simulink model "X31dynamics_03_controller_GainS_MG_old"  (R2014b)
settings: Solver=ode45  StartTime=0.0  StopTime=30  FixedStep=0.01  RelTol=1e-3
InitFcn:
  | X31dynamics_03_controller_GainS_MG_init
values from neighbouring files (symbols this model uses):
  X31_controller = evalin('base','X31_controller')    [X31dynamics_03_controller_MG_iter_3_2_9_10.m]
undefined symbols (not defined in the file or in its folder): sigbuilder_block, X31_initC, X31_MnvrGen
libraries: simulink x9, QuaternionLib x5
settings Model: Creator=Ewing  LastModifiedBy=5909
settings SolverCC: AlgebraicLoopSolver=LineSearch
settings DataIOCC: SaveOutput=off  SaveTime=off
settings OptimizationCC: InlineParams=on  InlineInvariantSignals=on  EfficientFloat2IntCast=on
settings DebuggingCC: UnderspecifiedInitializationDetection=Classic  MergeDetectMultiDrivingBlocksExec=none  UniqueDataStoreMsg=error  StateNameClashWarn=warning
settings ModelReferenceCC: ModelReferencePassRootInputsByReference=off

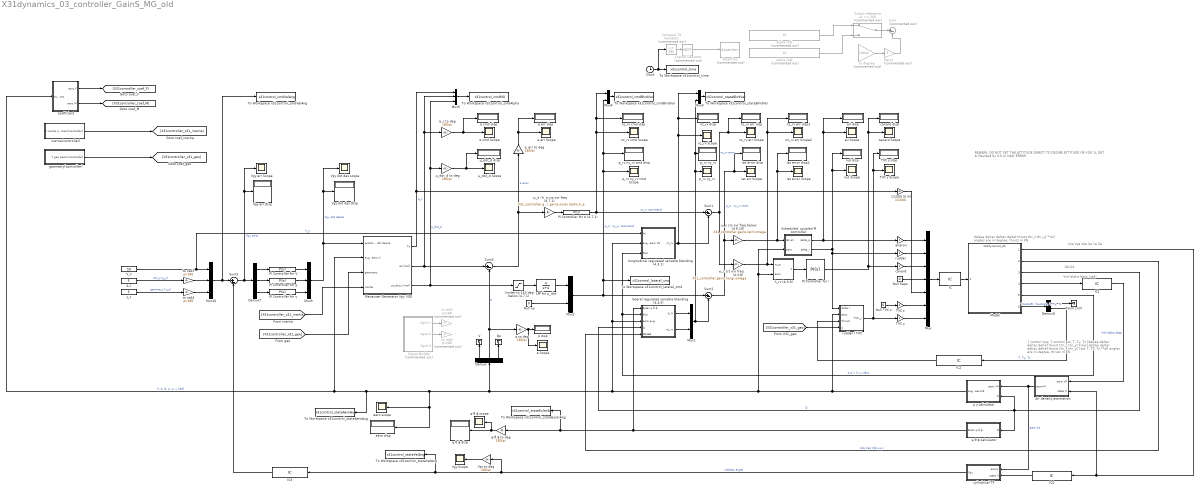
== system X31dynamics_03_controller_GainS_MG_old ==
  note: REMARK: DO NOT SET THE ATTITUDE DIRECT TO DESIRE ATTITUDE
      | OR YOU"LL GET A 'Devided by 0.0 or NaN' ERROR
  note: Q0-Q3
  note: Vxe Vye Vze
      | Xe   Ye   Ze
  note: deltaa deltar deltac deltaf thrust thr_z thr_y]
      | **all angles are in degree, thrust in KN
  note: Vinf alpha beta (rad)
  note: 7 contorl raw, 7 control act, T, Ty, Tz
      | [deltaa deltar deltac deltaf thrust thr_z thr_y] 7raw
      | [deltaa deltar deltac deltaf thrust thr_z thr_y] 7act
      | T, Ty, Tz
      | **all angles are in degree, thrust in KN
  1/1000 (K N) : Gain  Gain=1/1000
  Air density estimation : Subsystem
  Assertion : Assertion  Commented=on  AssertionFailFcn=|  StopWhenAssertionFail=off
      | set_param(bdroot,'SimulationCommand','pause'),
      | disp(sprintf('\nSimulation paused.'))
  Clock : Clock
  Compare To Constant : simulink/Logic and Bit Operations/Compare To Constant  Commented=on  relop=>=  const=180  OutDataTypeStr=boolean
  Demux : Demux  Outputs=[1 1 4]
  Demux7 : Demux  Outputs=3
  Demux9 : Demux  Outputs=[14 3]
  Gain1 : Gain  Commented=on  Gain=3
  IC : InitialCondition  Value=[ 0.0001 0.0001 00001 0 X31_initC.thrust 0 0.0001]
  IC1 : InitialCondition  Value=[50 0.01 0.01]
  IC2 : InitialCondition  Value=[X31_initC.thrust 0.00001 0]
  IC3 : InitialCondition  Value=[50 0 0]
  IC4 : InitialCondition  Value=[50 0 0 0.1 0.1 -0.1]
  LPF for μ_dot : TransferFcn  Numerator=[4]  Denominator=[1 4]
  Logical Operator : Logic  Commented=on  Operator=NOT  AllPortsSameDT=off  OutDataTypeStr=boolean
  Maneuver Generator Vχγ  NDI : Subsystem
  Model : ModelReference  ModelNameDialog=X31dynamics_03.slx  SimulationMode=Normal  ModelReferenceVersion=1.302  CopyOfModelName=X31dynamics_03.slx  DefaultDataLogging=on
  Mux : Mux  Inputs=7
  Mux{1..4} (4 alike) : Mux  Inputs=2
  Mux10 : Mux  Inputs=3
  Mux5 : Mux  Inputs=3
  Mux9 : Mux  Inputs=3
  Null TVC z : Constant  Value=0
  Null flaps : Constant  Value=0
  Null ny : Constant  Value=0
  PI Controller for V : simulink/Continuous/PID Controller  Controller=PI  TimeDomain=Continuous-time  SampleTime=-1  IntegratorMethod=Forward Euler  FilterMethod=Forward Euler  Form=Parallel  P=X31_MnvrGen.gains.vel.P_gain  I=X31_MnvrGen.gains.vel.I_gain  D=0  N=100  InitialConditionSource=internal  InitialConditionForIntegrator=0  InitialConditionForFilter=0  ExternalReset=none  LimitOutput=off  UpperSaturationLimit=inf  LowerSaturationLimit=-inf  LinearizeAsGain=on  AntiWindupMode=none  Kb=1  TrackingMode=off  Kt=1  PParamMin=[]  PParamMax=[]  IParamMin=[]  IParamMax=[]  DParamMin=[]  DParamMax=[]  NParamMin=[]  NParamMax=[]  KbParamMin=[]  KbParamMax=[]  KtParamMin=[]  KtParamMax=[]  POutMin=[]  POutMax=[]  IOutMin=[]  IOutMax=[]  DOutMin=[]  DOutMax=[]  NOutMin=[]  NOutMax=[]  KbOutMin=[]  KbOutMax=[]  KtOutMin=[]  KtOutMax=[]  IntegratorOutMin=[]  IntegratorOutMax=[]  FilterOutMin=[]  FilterOutMax=[]  SumOutMin=[]  SumOutMax=[]  SumI1OutMin=[]  SumI1OutMax=[]  SumI2OutMin=[]  SumI2OutMax=[]  SumI3OutMin=[]  SumI3OutMax=[]  SumDOutMin=[]  SumDOutMax=[]  SaturationOutMin=[]  SaturationOutMax=[]  IntegratorContinuousStateAttributes=''  IntegratorStateMustResolveToSignalObject=off  IntegratorRTWStateStorageClass=Auto  FilterContinuousStateAttributes=''  FilterStateMustResolveToSignalObject=off  FilterRTWStateStorageClass=Auto  DifferentiatorICPrevScaledInput=0  DifferentiatorOutMin=[]  DifferentiatorOutMax=[]  UseFilter=on
  PI Controller for r : simulink/Continuous/PID Controller  Controller=PI  TimeDomain=Continuous-time  SampleTime=-1  IntegratorMethod=Forward Euler  FilterMethod=Forward Euler  Form=Parallel  P=X31_controller.gains.longi.P_gain  I=X31_controller.gains.longi.I_gain  D=0  N=100  InitialConditionSource=internal  InitialConditionForIntegrator=0  InitialConditionForFilter=0  ExternalReset=none  LimitOutput=off  UpperSaturationLimit=inf  LowerSaturationLimit=-inf  LinearizeAsGain=on  AntiWindupMode=none  Kb=1  TrackingMode=off  Kt=1  PParamMin=[]  PParamMax=[]  IParamMin=[]  IParamMax=[]  DParamMin=[]  DParamMax=[]  NParamMin=[]  NParamMax=[]  KbParamMin=[]  KbParamMax=[]  KtParamMin=[]  KtParamMax=[]  POutMin=[]  POutMax=[]  IOutMin=[]  IOutMax=[]  DOutMin=[]  DOutMax=[]  NOutMin=[]  NOutMax=[]  KbOutMin=[]  KbOutMax=[]  KtOutMin=[]  KtOutMax=[]  IntegratorOutMin=[]  IntegratorOutMax=[]  FilterOutMin=[]  FilterOutMax=[]  SumOutMin=[]  SumOutMax=[]  SumI1OutMin=[]  SumI1OutMax=[]  SumI2OutMin=[]  SumI2OutMax=[]  SumI3OutMin=[]  SumI3OutMax=[]  SumDOutMin=[]  SumDOutMax=[]  SaturationOutMin=[]  SaturationOutMax=[]  IntegratorContinuousStateAttributes=''  IntegratorStateMustResolveToSignalObject=off  IntegratorRTWStateStorageClass=Auto  FilterContinuousStateAttributes=''  FilterStateMustResolveToSignalObject=off  FilterRTWStateStorageClass=Auto  DifferentiatorICPrevScaledInput=0  DifferentiatorOutMin=[]  DifferentiatorOutMax=[]  UseFilter=on
  PI Controller for α (4.7.1) : simulink/Continuous/PID Controller  Controller=PI  TimeDomain=Continuous-time  SampleTime=-1  IntegratorMethod=Forward Euler  FilterMethod=Forward Euler  Form=Parallel  P=X31_controller.gains.outer.alpha.P_gain  I=X31_controller.gains.outer.alpha.I_gain  D=0  N=100  InitialConditionSource=internal  InitialConditionForIntegrator=0  InitialConditionForFilter=0  ExternalReset=none  LimitOutput=off  UpperSaturationLimit=inf  LowerSaturationLimit=-inf  LinearizeAsGain=on  AntiWindupMode=none  Kb=1  TrackingMode=off  Kt=1  PParamMin=[]  PParamMax=[]  IParamMin=[]  IParamMax=[]  DParamMin=[]  DParamMax=[]  NParamMin=[]  NParamMax=[]  KbParamMin=[]  KbParamMax=[]  KtParamMin=[]  KtParamMax=[]  POutMin=[]  POutMax=[]  IOutMin=[]  IOutMax=[]  DOutMin=[]  DOutMax=[]  NOutMin=[]  NOutMax=[]  KbOutMin=[]  KbOutMax=[]  KtOutMin=[]  KtOutMax=[]  IntegratorOutMin=[]  IntegratorOutMax=[]  FilterOutMin=[]  FilterOutMax=[]  SumOutMin=[]  SumOutMax=[]  SumI1OutMin=[]  SumI1OutMax=[]  SumI2OutMin=[]  SumI2OutMax=[]  SumI3OutMin=[]  SumI3OutMax=[]  SumDOutMin=[]  SumDOutMax=[]  SaturationOutMin=[]  SaturationOutMax=[]  IntegratorContinuousStateAttributes=''  IntegratorStateMustResolveToSignalObject=off  IntegratorRTWStateStorageClass=Auto  FilterContinuousStateAttributes=''  FilterStateMustResolveToSignalObject=off  FilterRTWStateStorageClass=Auto  DifferentiatorICPrevScaledInput=0  DifferentiatorOutMin=[]  DifferentiatorOutMax=[]  UseFilter=on
  PI Controller for γ : simulink/Continuous/PID Controller  Controller=PI  TimeDomain=Continuous-time  SampleTime=-1  IntegratorMethod=Forward Euler  FilterMethod=Forward Euler  Form=Parallel  P=X31_MnvrGen.gains.gamma.P_gain  I=X31_MnvrGen.gains.gamma.P_gain  D=0  N=100  InitialConditionSource=internal  InitialConditionForIntegrator=0  InitialConditionForFilter=0  ExternalReset=none  LimitOutput=off  UpperSaturationLimit=inf  LowerSaturationLimit=-inf  LinearizeAsGain=on  AntiWindupMode=none  Kb=1  TrackingMode=off  Kt=1  PParamMin=[]  PParamMax=[]  IParamMin=[]  IParamMax=[]  DParamMin=[]  DParamMax=[]  NParamMin=[]  NParamMax=[]  KbParamMin=[]  KbParamMax=[]  KtParamMin=[]  KtParamMax=[]  POutMin=[]  POutMax=[]  IOutMin=[]  IOutMax=[]  DOutMin=[]  DOutMax=[]  NOutMin=[]  NOutMax=[]  KbOutMin=[]  KbOutMax=[]  KtOutMin=[]  KtOutMax=[]  IntegratorOutMin=[]  IntegratorOutMax=[]  FilterOutMin=[]  FilterOutMax=[]  SumOutMin=[]  SumOutMax=[]  SumI1OutMin=[]  SumI1OutMax=[]  SumI2OutMin=[]  SumI2OutMax=[]  SumI3OutMin=[]  SumI3OutMax=[]  SumDOutMin=[]  SumDOutMax=[]  SaturationOutMin=[]  SaturationOutMax=[]  IntegratorContinuousStateAttributes=''  IntegratorStateMustResolveToSignalObject=off  IntegratorRTWStateStorageClass=Auto  FilterContinuousStateAttributes=''  FilterStateMustResolveToSignalObject=off  FilterRTWStateStorageClass=Auto  DifferentiatorICPrevScaledInput=0  DifferentiatorOutMin=[]  DifferentiatorOutMax=[]  UseFilter=on
  PI Controller for χ : simulink/Continuous/PID Controller  Controller=PI  TimeDomain=Continuous-time  SampleTime=-1  IntegratorMethod=Forward Euler  FilterMethod=Forward Euler  Form=Parallel  P=X31_MnvrGen.gains.chi.P_gain  I=X31_MnvrGen.gains.chi.I_gain  D=0  N=100  InitialConditionSource=internal  InitialConditionForIntegrator=0  InitialConditionForFilter=0  ExternalReset=none  LimitOutput=off  UpperSaturationLimit=inf  LowerSaturationLimit=-inf  LinearizeAsGain=on  AntiWindupMode=none  Kb=1  TrackingMode=off  Kt=1  PParamMin=[]  PParamMax=[]  IParamMin=[]  IParamMax=[]  DParamMin=[]  DParamMax=[]  NParamMin=[]  NParamMax=[]  KbParamMin=[]  KbParamMax=[]  KtParamMin=[]  KtParamMax=[]  POutMin=[]  POutMax=[]  IOutMin=[]  IOutMax=[]  DOutMin=[]  DOutMax=[]  NOutMin=[]  NOutMax=[]  KbOutMin=[]  KbOutMax=[]  KtOutMin=[]  KtOutMax=[]  IntegratorOutMin=[]  IntegratorOutMax=[]  FilterOutMin=[]  FilterOutMax=[]  SumOutMin=[]  SumOutMax=[]  SumI1OutMin=[]  SumI1OutMax=[]  SumI2OutMin=[]  SumI2OutMax=[]  SumI3OutMin=[]  SumI3OutMax=[]  SumDOutMin=[]  SumDOutMax=[]  SaturationOutMin=[]  SaturationOutMax=[]  IntegratorContinuousStateAttributes=''  IntegratorStateMustResolveToSignalObject=off  IntegratorRTWStateStorageClass=Auto  FilterContinuousStateAttributes=''  FilterStateMustResolveToSignalObject=off  FilterRTWStateStorageClass=Auto  DifferentiatorICPrevScaledInput=0  DifferentiatorOutMin=[]  DifferentiatorOutMax=[]  UseFilter=on
  "Scheduled, coupled PI controller" : Subsystem
  Signal Builder : Subsystem  Tag=STV Subsys  Commented=on  LoadFcn=sigbuilder_block('load');  StartFcn=sigbuilder_block('start');  StopFcn=sigbuilder_block('stop');  ClipboardFcn=sigbuilder_block('clipboard');  mask(Sigbuilder block){}
      mask help: Simulink:masks:SigbuilderBlock_MD
      mask init:
      | if ~strcmp(get_param(bdroot(gcbh),'SimulationStatus'),'stopped') tuvar = sigbuilder_block('maskInit'); end
      settings: CopyFcn=sigbuilder_block('copy');  DeleteFcn=sigbuilder_block('delete');  ModelCloseFcn=sigbuilder_block('modelClose');  PreSaveFcn=sigbuilder_block('preSave');  PauseFcn=sigbuilder_block('pause');  ContinueFcn=sigbuilder_block('continue');  NameChangeFcn=sigbuilder_block('namechange');  OpenFcn=sigbuilder_block('open',[437.6 199.2 550.4 400 ]);  CloseFcn=sigbuilder_block('close');
      mask Display: plot(0, 0, 100, 100,[2, 2, 32, 32, 2], [68, 8, 8, 68, 68],[32, 2], [38, 38], [32, 19, 2],[53, 60, 44], [32, 17, 17, 2],[16, 16, 31, 31]);txt = getActiveGroup(gcbh);text(2, 100, txt,'verticalAlignment', 'top');
  Sum : Sum  Commented=on  Inputs=|+-
  Sum{1..3,5} (4 alike) : Sum  Inputs=|+-
  Switch reference : Switch  Commented=on  Threshold=200
  TVC y : Gain
  TVC y Scope : Scope
      settings: SaveName=ScopeData13
  TVC y disp : Display
  TVC z : Gain
  Term cntrl : Terminator
  To Workspace x31control_cmdAlpha : ToWorkspace  VariableName=x31control_cmdMG  SaveFormat=Timeseries  SampleTime=-1
  To Workspace x31control_cmdBlndVar : ToWorkspace  VariableName=x31control_cmdBlndVar  SaveFormat=Timeseries  SampleTime=-1
  To Workspace x31control_cmdVelAng : ToWorkspace  VariableName=x31control_cmdVelAng  SaveFormat=Timeseries  SampleTime=-1
  To Workspace x31control_lateral_cmd : ToWorkspace  VariableName=x31control_lateral_cmd  SaveFormat=Timeseries  SampleTime=-1
  To Workspace x31control_stateAeroAug : ToWorkspace  VariableName=x31control_stateAeroAug  SaveFormat=Timeseries  SampleTime=-1
  To Workspace x31control_stateBlndVar : ToWorkspace  VariableName=x31control_stateBlndVar  SaveFormat=Timeseries  SampleTime=-1
  To Workspace x31control_stateEulerAng : ToWorkspace  VariableName=x31control_stateEulerAng  SaveFormat=Timeseries  SampleTime=-1
  To Workspace x31control_stateVelAng : ToWorkspace  VariableName=x31control_stateVelAng  SaveFormat=Timeseries  SampleTime=-1
  To Workspace x31control_time : ToWorkspace  VariableName=x31control_time  SaveFormat=Timeseries  SampleTime=-1
  V : Terminator
  V_c : Constant  Value=50
  Vχγ Scope : Scope
      settings: ShowLegends=on  TimeRange=30  YMin=-1000  YMax=6000  SaveName=ScopeData18
  Vχγ dot des Disp : Display
  Vχγ dot des scope : Scope
      settings: TickLabels=on  ShowLegends=on  SaveName=ScopeData15
  Vχγ err Disp : Display
  Vχγ err Scope : Scope
      settings: TimeRange=3.005065038857998  YMin=2.02995391705069  YMax=6.02995391705069  SaveName=ScopeData14
  Vχγ to deg : Gain  Gain=180/pi
  aero disp : Display
  aero scope : Scope
      settings: ShowLegends=on  YMin=-1000  YMax=6000  SaveName=ScopeData8
  ail Scope : Scope
      settings: SaveName=ScopeData11
  ail disp : Display
  aileron : Gain
  alpha ref1 : Constant  Commented=on  Value=10
  alpha ref2 : Constant  Commented=on  Value=10
  canard : Gain
  canard Scope : Scope
      settings: SaveName=ScopeData12
  canard disp : Display
  coefficient : Subsystem
  cylindrical TF : Subsystem
  geometry(controller) : Subsystem
  h_rv (4.3.9) : Subsystem
  inertia(controller) : Subsystem
  lat err Scope : Scope
      settings: SaveName=ScopeData5
  lat error Scope : Scope
      settings: SaveName=ScopeData9
  lat error disp : Display
  lat error disp2 : Display
  lateral regulated variable blending (4.4.5) : Subsystem
  limiter to 143 deg below (4.7.1) : Saturate  UpperLimit=143 * pi / 180  LowerLimit=-143 * pi / 180
  longitudinal regulated variable blending (4.3.1) : Subsystem
  nz_rv Scope : Scope
      settings: SaveName=ScopeData16
  nz_rv cmd Scope : Scope
      settings: SaveName=ScopeData2
  nz_rv cmd disp : Display
  nz_rv disp : Display
  nz_rv err Scope : Scope
      settings: SaveName=ScopeData7
  nz_rv err Scope2 : Scope
      settings: SaveName=ScopeData10
  nz_rv err disp : Display
  nz_rv err disp2 : Display
  p_rv ny_rv : Display
  "p_rv ny_rv " : Scope
      settings: SaveName=ScopeData6
  p_rv ny_rv cmd Scope : Scope
      settings: SaveName=ScopeData4
  p_rv ny_rv cmd disp : Display
  rud Scope : Scope
      settings: SaveName=ScopeData17
  rud disp : Display
  rudder : Gain
  rudder / TVC : Subsystem
  to degree : Gain  Commented=on  Gain=180/pi
  to rad1 : Gain  Commented=on  Gain=pi/180
  to rad2 : Gain  Commented=on  Gain=pi/180
  to rad3 : Gain  Gain=pi/180
  to rad4 : Gain  Gain=pi/180
  α Scope : Scope
      settings: SaveName=ScopeData20
  α cmd Scope : Scope
  α cmd disp : Display
  α disp : Display
  α err Scope : Scope
  α err disp : Display
  α to deg : Gain  Gain=180/pi
  α_c to deg : Gain  Gain=180/pi
  α_err to deg : Gain  Gain=180/pi
  βρ : Terminator
  γ_c : Constant  Value=5
  μ γ calculator : Subsystem
  μ_dot_d Scope : Scope
      settings: SaveName=ScopeData3
  μ_dot_d disp : Display
  μ_dot_d to deg : Gain  Gain=180/pi
  χ_c : Constant  Value=5
  ψ θ ϕ calculator : Subsystem
  ψ θ ϕ disp : Display
  ψ θ ϕ scope : Scope
      settings: ShowLegends=on  TimeRange=30  YMin=-20  YMax=160  SaveName=ScopeData19
  ψ θ ϕ to deg : Gain  Gain=180/pi
  ω_a / h_a crs ovr freq (4.7.1) : Gain  Gain=X31_controller.gains.outer.alpha.omega / X31_controller.gains.outer.alpha.h_a
  ω_c crs ovr freq (4.3.8) : Gain  Gain=X31_controller.gains.longi.omega
  ω_c crs ovr freq below (4.6.10) : Gain  Gain=X31_controller.gains.latrl.omega
  wires:
  Null flaps/1 -> Mux/4
  rudder/1 -> Mux/2
  canard/1 -> Mux/3
  Mux/1 -> IC/1
  IC/1 -> Model/1
  alpha ref1/1 -> Switch reference/1
  alpha ref2/1 -> Switch reference/3
  Clock/1 -> Compare To Constant/1, To Workspace x31control_time/1
  aileron/1 -> Mux/1
  Model/4 -> IC1/1
  Switch reference/1 -> Sum/1
  to degree/1 -> Gain1/1
  Maneuver Generator Vχγ  NDI/1(Tc) -> Mux5/1, 1/1000 (K N)/1
  Gain1/1 -> Sum/2
  TVC z/1 -> Mux/6
  TVC y/1 -> Mux/7
  [X31controller_x31_geo] -> rudder / TVC/4(geometry)
  Null TVC z/1 -> TVC z/1
  rudder / TVC/1(TVC_y) -> TVC y/1, TVC y Scope/1, TVC y disp/1
  Sum1/1 -> ω_c crs ovr freq (4.3.8)/1, nz_rv err disp/1, nz_rv err Scope/1  "nz_rv error"
  Model/2 -> lateral regulated variable blending (4.4.5)/5(stateB)  "Vxb Vyb Vzb p q r"
  coefficient/1(aero F) -> [X31controller_coef_F]
  coefficient/2(aero M) -> [X31controller_coef_M]
  Maneuver Generator Vχγ  NDI/2(αc (rad)) -> α_c to deg/1, Mux5/2, Sum3/1  "α_c"
  μ γ calculator/1(aug. aeroV6) -> To Workspace x31control_stateAeroAug/1, coefficient/1(aug. aero), Maneuver Generator Vχγ  NDI/2(aug. aero V), aero scope/1, aero disp/1, Demux/1, longitudinal regulated variable blending (4.3.1)/2(aug. aero V6), lateral regulated variable blending (4.4.5)/3(aero aug.), "Scheduled, coupled PI controller"/2(aero), h_rv (4.3.9)/2(aero), rudder / TVC/2(aero)  "V, α, β, ρ, μ, γ (rad)"
  Sum3/1 -> α_err to deg/1, ω_a / h_a crs ovr freq (4.7.1)/1  "α error"
  Maneuver Generator Vχγ  NDI/3(μc_dot_c (rad)) -> μ_dot_d to deg/1, Mux5/3, limiter to 143 deg below (4.7.1)/1  "μ_dot_d"
  Model/3 -> ψ θ ϕ calculator/1(Q), lateral regulated variable blending (4.4.5)/4(Q), μ γ calculator/2(Q)  "Q"
  Demux9/2 -> IC2/1  "T, Ty, Tz"
  Demux/1 -> V/1
  Demux/3 -> βρ/1
  IC1/1 -> Air density estimation/1(aero V3)  "Vinf alpha beta"
  Demux9/1 -> Term cntrl/1
  Model/6 -> Demux9/1  "7controR, 7controlA, T, Ty, Tz"
  Model/5 -> longitudinal regulated variable blending (4.3.1)/3(IMU), lateral regulated variable blending (4.4.5)/2(IMU)  "p q r, (x y z)acc"
  longitudinal regulated variable blending (4.3.1)/1(nz_rv) -> Sum1/2, nz_rv Scope/1, Mux3/1, nz_rv disp/1
  ω_c crs ovr freq (4.3.8)/1 -> h_rv (4.3.9)/1(nz_e), nz_rv err Scope2/1, nz_rv err disp2/1
  PI Controller for α (4.7.1)/1 -> Sum1/1, nz_rv cmd Scope/1, Mux4/1, nz_rv cmd disp/1  "nz_rv command"
  h_rv (4.3.9)/1(1 /h_rv) -> PI Controller for r/1
  ψ θ ϕ calculator/1(Eular ψ θ ϕ) -> To Workspace x31control_stateEulerAng/1, ψ θ ϕ to deg/1, lateral regulated variable blending (4.4.5)/1(Eular ψ θ ϕ)
  "Scheduled, coupled PI controller"/2(delta_r) -> rudder/1, rudder / TVC/1(delta r), rud disp/1, rud Scope/1
  lateral regulated variable blending (4.4.5)/1(p_rv) -> Mux1/1
  lateral regulated variable blending (4.4.5)/2(ny_rv) -> Mux1/2
  Mux2/1 -> Sum2/1, Mux4/2, p_rv ny_rv cmd disp/1, p_rv ny_rv cmd Scope/1, To Workspace x31control_lateral_cmd/1  "p_rv  ny_rv command"
  Mux1/1 -> Sum2/2, Mux3/2, p_rv ny_rv/1, "p_rv ny_rv "/1
  Sum2/1 -> lat error disp/1, lat err Scope/1, ω_c crs ovr freq below (4.6.10)/1  "p_rv  ny_rv error"
  ω_c crs ovr freq below (4.6.10)/1 -> "Scheduled, coupled PI controller"/1(lat err), lat error disp2/1, lat error Scope/1
  "Scheduled, coupled PI controller"/1(delta_a) -> ail disp/1, ail Scope/1, aileron/1
  Null ny/1 -> Mux2/2
  limiter to 143 deg below (4.7.1)/1 -> LPF for μ_dot/1
  ω_a / h_a crs ovr freq (4.7.1)/1 -> PI Controller for α (4.7.1)/1
  LPF for μ_dot/1 -> Mux2/1
  IC2/1 -> rudder / TVC/3(Thrust)
  geometry(controller)/1(7 geo param(controller)) -> [X31controller_x31_geo]
  inertia(controller)/1(7 inertia param(controller)) -> [X31controller_x31_inertia]
  Mux10/1 -> To Workspace x31control_cmdVelAng/1, Sum5/1
  Sum5/1 -> Demux7/1, Vχγ err Disp/1, Vχγ err Scope/1  "Vχγ error"
  Demux7/3 -> PI Controller for γ/1
  Demux7/2 -> PI Controller for χ/1
  Demux7/1 -> PI Controller for V/1
  PI Controller for γ/1 -> Mux9/3
  PI Controller for χ/1 -> Mux9/2
  PI Controller for V/1 -> Mux9/1
  Mux9/1 -> Maneuver Generator Vχγ  NDI/1(positionVχγ dot desire), Vχγ dot des scope/1, Vχγ dot des Disp/1  "Vχγ dot desire"
  V_c/1 -> longitudinal regulated variable blending (4.3.1)/1(Vc), Mux10/1  "V_c"
  χ_c/1 -> to rad3/1  "Chi_c (χ_c)"
  γ_c/1 -> to rad4/1  "gamma_c (γ_c)"
  to rad3/1 -> Mux10/2
  to rad4/1 -> Mux10/3
  Air density estimation/1(aeroV4) -> cylindrical TF/1(aeroV), μ γ calculator/1(aero V4)  "aero V4"
  cylindrical TF/1(Vχγ) -> To Workspace x31control_stateVelAng/1, IC3/1, Vχγ to deg/1  "velocity angle"
  Model/1 -> Air density estimation/2(state X), IC4/1
  Demux/2 -> Sum3/2, α to deg/1  "α"
  IC3/1 -> Sum5/2
  IC4/1 -> cylindrical TF/2(state X)
  PI Controller for r/1 -> canard Scope/1, canard disp/1, canard/1
  1/1000 (K N)/1 -> Mux/5
  Compare To Constant/1 -> Logical Operator/1
  Logical Operator/1 -> Assertion/1
  ψ θ ϕ to deg/1 -> ψ θ ϕ disp/1, ψ θ ϕ scope/1
  Vχγ to deg/1 -> Vχγ Scope/1
  [X31controller_x31_geo] -> Maneuver Generator Vχγ  NDI/3(geometry)
  [X31controller_x31_inertia] -> Maneuver Generator Vχγ  NDI/4(inertia)
  α to deg/1 -> α Scope/1, α disp/1
  Signal Builder/1(Signal 1) -> to rad1/1
  Signal Builder/2(Signal 2) -> to rad2/1
  α_c to deg/1 -> α cmd Scope/1, α cmd disp/1
  μ_dot_d to deg/1 -> μ_dot_d Scope/1, μ_dot_d disp/1
  Mux3/1 -> To Workspace x31control_stateBlndVar/1
  Mux4/1 -> To Workspace x31control_cmdBlndVar/1
  α_err to deg/1 -> α err disp/1, α err Scope/1
  Mux5/1 -> To Workspace x31control_cmdAlpha/1

== system X31dynamics_03_controller_GainS_MG_old/Air density estimation ==
  aero V3 : Inport
  state X : Inport  Port=2
  Mux : Mux  Inputs=2
  Terminator : Terminator
  air_density : Constant  Value=1.23
  aeroV4 : Outport
  wires:
  aero V3/1 -> Mux/1
  Mux/1 -> aeroV4/1
  air_density/1 -> Mux/2
  state X/1 -> Terminator/1

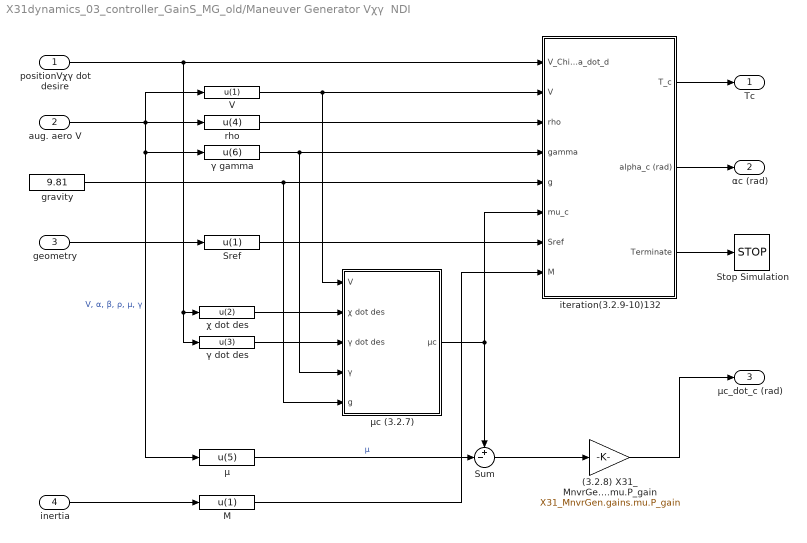
== system X31dynamics_03_controller_GainS_MG_old/Maneuver Generator Vχγ  NDI ==
  positionVχγ dot desire : Inport
  aug. aero V : Inport  Port=2
  geometry : Inport  Port=3
  inertia : Inport  Port=4
  (3.2.8) X31_MnvrGen.gains.mu.P_gain : Gain  Gain=X31_MnvrGen.gains.mu.P_gain
  M : Fcn  Expr=u(1)
  Sref : Fcn  Expr=u(1)
  Stop Simulation : Stop
  Sum : Sum  Inputs=+-|
  V : Fcn  Expr=u(1)
  gravity : Constant  Value=9.81
  iteration(3.2.9-10)132 : Subsystem
  rho : Fcn  Expr=u(4)
  γ dot des : Fcn  Expr=u(3)
  γ gamma : Fcn  Expr=u(6)
  μ : Fcn  Expr=u(5)
  μc (3.2.7) : Subsystem
  χ dot des : Fcn  Expr=u(2)
  Tc : Outport
  αc (rad) : Outport  Port=2
  μc_dot_c (rad) : Outport  Port=3
  wires:
  positionVχγ dot desire/1 -> γ dot des/1, χ dot des/1, iteration(3.2.9-10)132/1(V_Chi_Gamma_dot_d)
  aug. aero V/1 -> μ/1, γ gamma/1, V/1, rho/1  "V, α, β, ρ, μ, γ"
  μc (3.2.7)/1(μc) -> iteration(3.2.9-10)132/6(mu_c), Sum/1
  μ/1 -> Sum/2  "μ"
  Sum/1 -> (3.2.8) X31_MnvrGen.gains.mu.P_gain/1
  (3.2.8) X31_MnvrGen.gains.mu.P_gain/1 -> μc_dot_c (rad)/1
  iteration(3.2.9-10)132/2(alpha_c (rad)) -> αc (rad)/1
  iteration(3.2.9-10)132/1(T_c) -> Tc/1
  geometry/1 -> Sref/1
  inertia/1 -> M/1
  V/1 -> μc (3.2.7)/1(V), iteration(3.2.9-10)132/2(V)
  γ dot des/1 -> μc (3.2.7)/3(γ dot des)
  χ dot des/1 -> μc (3.2.7)/2(χ dot des)
  gravity/1 -> μc (3.2.7)/5(g), iteration(3.2.9-10)132/5(g)
  γ gamma/1 -> μc (3.2.7)/4(γ), iteration(3.2.9-10)132/4(gamma)
  rho/1 -> iteration(3.2.9-10)132/3(rho)
  iteration(3.2.9-10)132/3(Terminate) -> Stop Simulation/1
  Sref/1 -> iteration(3.2.9-10)132/7(Sref)
  M/1 -> iteration(3.2.9-10)132/8(M)

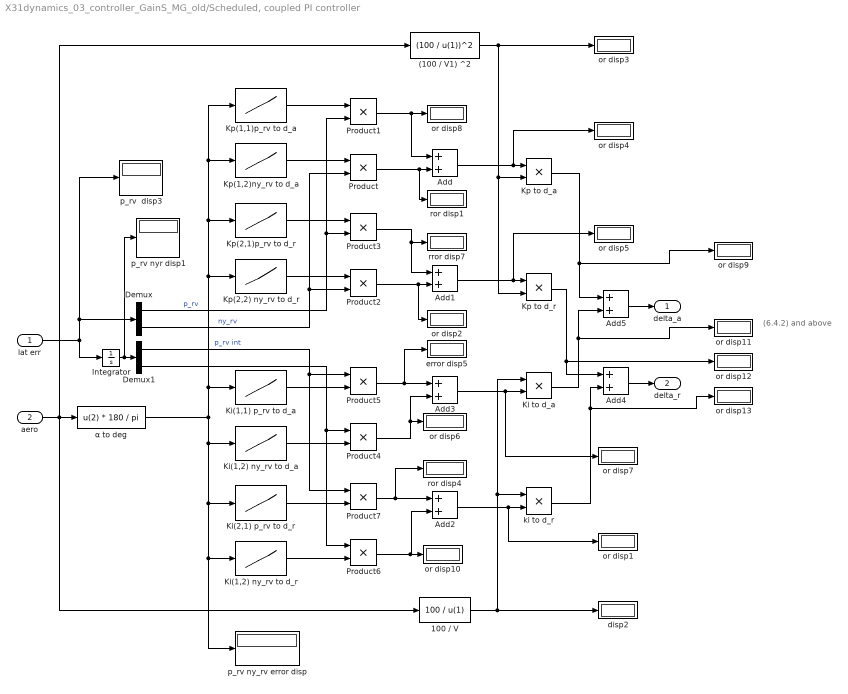
== system X31dynamics_03_controller_GainS_MG_old/Scheduled, coupled PI controller ==
  note: (6.4.2) and above
  lat err : Inport
  aero : Inport  Port=2
  " error disp5" : Display
  (100 / V1) ^2 : Fcn  Expr=(100 / u(1))^2
  100 / V : Fcn  Expr=100 / u(1)
  Add{,1..5} (6 alike) : Sum
  Demux : Demux  Outputs=2
  Demux1 : Demux  Outputs=2
  Integrator : Integrator
  Ki to d_a : Product
  Ki(1,1) p_rv to d_a : Lookup_n-D  NumberOfTableDimensions=1  BreakpointsForDimension1=X31_controller.gains.latrl.I_gain.mat1_1.alpha  Table=X31_controller.gains.latrl.I_gain.mat1_1.gain  ExtrapMethod=Clip  UseLastTableValue=on  InternalRulePriority=Speed  RndMeth=Simplest  InputSameDT=on
  Ki(1,2) ny_rv to d_a : Lookup_n-D  NumberOfTableDimensions=1  BreakpointsForDimension1=X31_controller.gains.latrl.I_gain.mat1_2.alpha  Table=X31_controller.gains.latrl.I_gain.mat1_2.gain  ExtrapMethod=Clip  UseLastTableValue=on  InternalRulePriority=Speed  RndMeth=Simplest  InputSameDT=on
  Ki(1,2) ny_rv to d_r : Lookup_n-D  NumberOfTableDimensions=1  BreakpointsForDimension1=X31_controller.gains.latrl.I_gain.mat2_2.alpha  Table=X31_controller.gains.latrl.I_gain.mat2_2.gain  ExtrapMethod=Clip  UseLastTableValue=on  InternalRulePriority=Speed  RndMeth=Simplest  InputSameDT=on
  Ki(2,1) p_rv to d_r : Lookup_n-D  NumberOfTableDimensions=1  BreakpointsForDimension1=X31_controller.gains.latrl.I_gain.mat2_1.alpha  Table=X31_controller.gains.latrl.I_gain.mat2_1.gain  ExtrapMethod=Clip  UseLastTableValue=on  InternalRulePriority=Speed  RndMeth=Simplest  InputSameDT=on
  Kp to d_a : Product
  Kp to d_r : Product
  Kp(1,1)p_rv to d_a : Lookup_n-D  NumberOfTableDimensions=1  BreakpointsForDimension1=X31_controller.gains.latrl.P_gain.mat1_1.alpha  Table=X31_controller.gains.latrl.P_gain.mat1_1.gain  ExtrapMethod=Clip  UseLastTableValue=on  InternalRulePriority=Speed  RndMeth=Simplest  InputSameDT=on
  Kp(1,2)ny_rv to d_a : Lookup_n-D  NumberOfTableDimensions=1  BreakpointsForDimension1=X31_controller.gains.latrl.P_gain.mat1_2.alpha  Table=X31_controller.gains.latrl.P_gain.mat1_2.gain  ExtrapMethod=Clip  UseLastTableValue=on  InternalRulePriority=Speed  RndMeth=Simplest  InputSameDT=on
  Kp(2,1)p_rv to d_r : Lookup_n-D  NumberOfTableDimensions=1  BreakpointsForDimension1=X31_controller.gains.latrl.P_gain.mat2_1.alpha  Table=X31_controller.gains.latrl.P_gain.mat2_1.gain  ExtrapMethod=Clip  UseLastTableValue=on  InternalRulePriority=Speed  RndMeth=Simplest  InputSameDT=on
  Kp(2,2) ny_rv to d_r : Lookup_n-D  NumberOfTableDimensions=1  BreakpointsForDimension1=X31_controller.gains.latrl.P_gain.mat2_2.alpha  Table=X31_controller.gains.latrl.P_gain.mat2_2.gain  ExtrapMethod=Clip  UseLastTableValue=on  InternalRulePriority=Speed  RndMeth=Simplest  InputSameDT=on
  Product{,1..7} (8 alike) : Product
  disp2 : Display
  ki to d_r : Product
  or disp{1..13} (13 alike) : Display
  p_rv  disp3 : Display
  p_rv ny_rv error disp : Display
  p_rv nyr disp1 : Display
  ror disp1 : Display
  ror disp4 : Display
  rror disp7 : Display
  α to deg : Fcn  Expr=u(2) * 180 / pi
  delta_a : Outport
  delta_r : Outport  Port=2
  wires:
  lat err/1 -> p_rv  disp3/1, Demux/1, Integrator/1
  Demux/2 -> Product/2, Product2/2  "ny_rv"
  Integrator/1 -> p_rv nyr disp1/1, Demux1/1
  Demux1/1 -> Product7/1, Product5/1  "p_rv int"
  Demux1/2 -> Product6/1, Product4/1
  aero/1 -> 100 / V/1, (100 / V1) ^2/1, α to deg/1
  Demux/1 -> Product1/2, Product3/2  "p_rv"
  Kp(1,2)ny_rv to d_a/1 -> Product/1
  Kp(1,1)p_rv to d_a/1 -> Product1/1
  Kp(2,1)p_rv to d_r/1 -> Product3/1
  Kp(2,2) ny_rv to d_r/1 -> Product2/1
  Ki(1,2) ny_rv to d_r/1 -> Product6/2
  Ki(2,1) p_rv to d_r/1 -> Product7/2
  Ki(1,1) p_rv to d_a/1 -> Product5/2
  α to deg/1 -> p_rv ny_rv error disp/1, Ki(1,2) ny_rv to d_r/1, Ki(2,1) p_rv to d_r/1, Ki(1,2) ny_rv to d_a/1, Kp(2,1)p_rv to d_r/1, Kp(1,1)p_rv to d_a/1, Kp(1,2)ny_rv to d_a/1, Kp(2,2) ny_rv to d_r/1, Ki(1,1) p_rv to d_a/1
  Product1/1 -> or disp8/1, Add/1
  Product/1 -> ror disp1/1, Add/2
  Product3/1 -> Add1/1, rror disp7/1
  Product2/1 -> or disp2/1, Add1/2
  Product5/1 -> Add3/1, " error disp5"/1
  Product7/1 -> Add2/1, ror disp4/1
  Product6/1 -> Add2/2, or disp10/1
  100 / V/1 -> Ki to d_a/1, ki to d_r/1, disp2/1
  Add2/1 -> or disp1/1, ki to d_r/2
  Add3/1 -> or disp7/1, Ki to d_a/2
  Add1/1 -> or disp5/1, Kp to d_r/1
  Add/1 -> or disp4/1, Kp to d_a/1
  Add4/1 -> delta_r/1
  Add5/1 -> delta_a/1
  Kp to d_a/1 -> or disp9/1, Add5/1
  Kp to d_r/1 -> Add4/1, or disp12/1
  ki to d_r/1 -> or disp13/1, Add4/2
  Ki(1,2) ny_rv to d_a/1 -> Product4/2
  Product4/1 -> Add3/2, or disp6/1
  (100 / V1) ^2/1 -> Kp to d_r/2, Kp to d_a/2, or disp3/1
  Ki to d_a/1 -> Add5/2, or disp11/1

== system X31dynamics_03_controller_GainS_MG_old/Signal Builder ==
  Demux : Demux  Tag=STV Demux  Outputs=3
  FromWs : FromWorkspace  Tag=STV FromWs  VariableName=tuvar  SampleTime=0
      SigBuilderData=|
      | common.afterFinalStr = 'Extrapolate'
      | common.sampleTime = 0
      | dataSet(1).timeRange = [0 30]
      | dataSet(1).name = 'Group 1'
      | dataSet(2).timeRange = [0 30]
      | dataSet(2).name = 'Group 2'
      | dataSet(3).timeRange = [0 30]
      | dataSet(3).name = 'Group 3'
      | dataSet(4).timeRange = [0 30]
      | dataSet(4).name = 'Group 4'
      | dataSet(5).timeRange = [0 30]
      | dataSet(5).name = 'Group 5'
      | sbobj.Groups(1).Name = 'Group 1'
      | sbobj.Groups(1).Signals(1).Name = 'Signal 1'
      | sbobj.Groups(1).Signals(1).XData = [0 5 5 25 25 30]
      | sbobj.Groups(1).Signals(1).YData = [10 10 30 30 10 10]
      | sbobj.Groups(1).Signals(2).Name = 'Signal 2'
      | sbobj.Groups(1).Signals(2).XData = [0 3 3 5 5 7 30]
      | sbobj.Groups(1).Signals(2).YData = [0 0 30 30 10 0 0]
      | sbobj.Groups(1).Signals(3).Name = 'Signal 3'
      | sbobj.Groups(1).Signals(3).XData = [0 1 1 20 20 30]
      | sbobj.Groups(1).Signals(3).YData = [80000 80000 120000 120000 80000 80000]
      | sbobj.Groups(1).TimeRange = [0 30]
      | sbobj.Groups(2).Name = 'Group 2'
      | sbobj.Groups(2).Signals(1).Name = 'Signal 1'
      | sbobj.Groups(2).Signals(1).XData = [0 4 15 30]
      | sbobj.Groups(2).Signals(1).YData = [-0.01 30 30 8.8]
      | sbobj.Groups(2).Signals(2).Name = 'Signal 2'
      | sbobj.Groups(2).Signals(2).XData = [0 0.625 1.25 1.875 2.5 3.125 3.75 4.375 5 5.625 6.25 6.875 7.5 8.125 8.75 9.375 10 10.625 11.25 11.875 12.5 13.125 13.75 14.375 15 15.625 16.25 16.875 17.5 18.125 18.75 19.375 20 20.625 21.25 21.875 22.5 23.125 23.75 24.375 25 25.625 26.25 26.875 27.5 28.125 28.75 29.375 30]
      | sbobj.Groups(2).Signals(2).YData = [0 14.1421356237 20 14.1421356237 2.44929359829e-15 -14.1421356237 -20 -14.1421356237 0 14.1421356237 20 14.1421356237 2.44929359829e-15 -14.1421356237 -20 -14.1421356237 0 14.1421356237 20 14.1421356237 2.44929359829e-15 -14.1421356237 -20 -14.1421356237 0 14.1421356237 20 14.1421356237 2.44929359829e-15 -14.1421356237 -20 -14.1421356237 0 14.1421356237 20 14.1421356237 2.44929359829e-15 -14.1421356237 -20 -14.1421356237 0 14.1421356237 20 14.1421356237 2.44929359829e-15 -14.1421356237 -20 -14.1421356237 0]
      | sbobj.Groups(2).Signals(3).Name = 'Signal 3'
      | sbobj.Groups(2).Signals(3).XData = [0 30]
      | sbobj.Groups(2).Signals(3).YData = [60 60]
      | sbobj.Groups(2).TimeRange = [0 30]
      | sbobj.Groups(3).Name = 'Group 3'
      | sbobj.Groups(3).Signals(1).Name = 'Signal 1'
      | sbobj.Groups(3).Signals(1).XData = [0 5 10 25 30]
      | sbobj.Groups(3).Signals(1).YData = [10 10 10 10 10]
      | sbobj.Groups(3).Signals(2).Name = 'Signal 2'
      | sbobj.Groups(3).Signals(2).XData = [0 3 3 9 9 30]
      | sbobj.Groups(3).Signals(2).YData = [0 0 30 30 0 0]
      | sbobj.Groups(3).Signals(3).Name = 'Signal 3'
      | sbobj.Groups(3).Signals(3).XData = [0 1 20 30]
      | sbobj.Groups(3).Signals(3).YData = [80000 80000 80000 80000]
      | sbobj.Groups(3).TimeRange = [0 30]
      | sbobj.Groups(4).Name = 'Group 4'
      | sbobj.Groups(4).Signals(1).Name = 'Signal 1'
      | sbobj.Groups(4).Signals(1).XData = [0 5 5 25 25 30]
      | sbobj.Groups(4).Signals(1).YData = [10 10 30 30 10 10]
      | sbobj.Groups(4).Signals(2).Name = 'Signal 2'
      | sbobj.Groups(4).Signals(2).XData = [0 3 3 8 8 9 30]
      | sbobj.Groups(4).Signals(2).YData = [0 0 30 30 10 0 0]
      | sbobj.Groups(4).Signals(3).Name = 'Signal 3'
      | sbobj.Groups(4).Signals(3).XData = [0 1 1 20 20 30]
      | sbobj.Groups(4).Signals(3).YData = [80000 80000 120000 120000 80000 80000]
      | sbobj.Groups(4).TimeRange = [0 30]
      | sbobj.Groups(5).Name = 'Group 5'
      | sbobj.Groups(5).Signals(1).Name = 'Signal 1'
      | sbobj.Groups(5).Signals(1).XData = [0 5 5 25 25 30]
      | sbobj.Groups(5).Signals(1).YData = [10 10 20 20 10 10]
      | sbobj.Groups(5).Signals(2).Name = 'Signal 2'
      | sbobj.Groups(5).Signals(2).XData = [0 3 3 5 5 7 30]
      | sbobj.Groups(5).Signals(2).YData = [0 0 30 30 10 0 0]
      | sbobj.Groups(5).Signals(3).Name = 'Signal 3'
      | sbobj.Groups(5).Signals(3).XData = [0 1 1 20 20 30]
      | sbobj.Groups(5).Signals(3).YData = [80000 80000 120000 120000 80000 80000]
      | sbobj.Groups(5).TimeRange = [0 30]
  Signal 1 : Outport  Tag=STV Outport
  Signal 2 : Outport  Tag=STV Outport  Port=2
  Signal 3 : Outport  Tag=STV Outport  Port=3
  wires:
  Demux/1 -> Signal 1/1
  FromWs/1 -> Demux/1
  Demux/2 -> Signal 2/1
  Demux/3 -> Signal 3/1

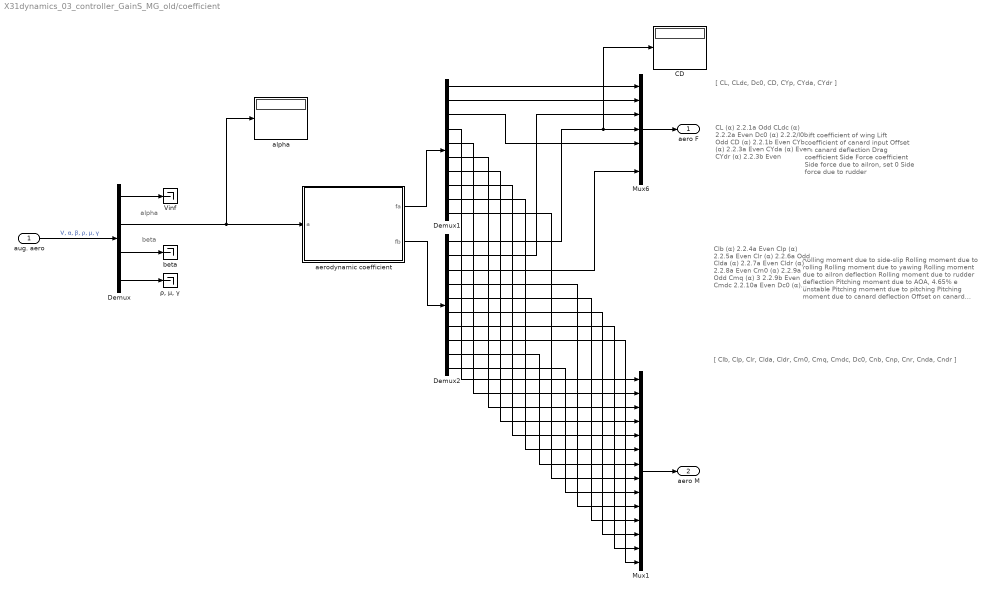
== system X31dynamics_03_controller_GainS_MG_old/coefficient ==
  note: Rolling moment due to side-slip
      | Rolling moment due to rolling
      | Rolling moment due to yawing
      | Rolling moment due to ailron deflection
      | Rolling moment due to rudder deflection
      |
      | Pitching moment due to AOA, 4.65% e unstable
      | Pitching moment due to pitching
      | Pitching moment due to canard deflection
      | Offset on canard deflection
      |
      | Yawing moment due to side-slip
      | Yawing moment due to rolling
      | Yawing moment due to yawing
      | Yawing moment due to ailron deflection
      | Yawing moment due to rudder deflection
  note: Lift coefficient of wing
      | Lift coefficient of canard input
      | Offset on canard deflection
      | Drag coefficient
      | Side Force coefficient
      | Side force due to ailron, set 0
      | Side force due to rudder
  note: Clb    (α) 2.2.4a Even
      | Clp    (α) 2.2.5a Even
      | Clr     (α) 2.2.6a Odd
      | Clda  (α) 2.2.7a Even
      | Cldr   (α) 2.2.8a Even
      |
      | Cm0  (α) 2.2.9a Odd
      | Cmq  (α) 3 2.2.9b Even
      | Cmdc      2.2.10a Even
      | Dc0   (α) 2.2.2/10b Odd
      |
      | Cnb  (α) 2.2.4b Even
      | Cnp  (α) 2.2.5b Odd
      | Cnr   (α) 2.2.6b Even
      | Cnda(α) 2.2.7b Even
      | Cndr (α) 2.2.8b Even
  note: CL     (α) 2.2.1a Odd
      | CLdc (α)  2.2.2a Even
      | Dc0   (α)  2.2.2/l0b Odd
      | CD     (α)  2.2.1b Even
      | CYb   (α) 2.2.3a Even
      | CYda (α)            Even
      | CYdr  (α) 2.2.3b Even
  note: beta
  note: alpha
  note: [ CL, CLdc, Dc0, CD, CYp, CYda, CYdr ]
  note: [ Clb, Clp, Clr, Clda, Cldr, Cm0, Cmq, Cmdc, Dc0, Cnb, Cnp, Cnr, Cnda, Cndr ]
  aug. aero : Inport
  CD : Display
  Demux : Demux  Outputs=[1 1 1 3]
  Demux1 : Demux  Outputs=10
  Demux2 : Demux  Outputs=10
  Mux1 : Mux  Inputs=14
  Mux6 : Mux  Inputs=7
  Vinf : Terminator
  aerodynamic coefficient : MATLAB Function  TreatAsAtomicUnit=on
  alpha : Display
  beta : Terminator
  "ρ, μ, γ" : Terminator
  aero F : Outport
  aero M : Outport  Port=2
  wires:
  Mux6/1 -> aero F/1
  aug. aero/1 -> Demux/1  "V, α, β, ρ, μ, γ"
  Demux/1 -> Vinf/1
  Mux1/1 -> aero M/1
  aerodynamic coefficient/1(fa) -> Demux1/1
  aerodynamic coefficient/2(fb) -> Demux2/1
  Demux1/1 -> Mux6/1
  Demux1/2 -> Mux6/2
  Demux2/2 -> Mux6/3
  Demux2/1 -> CD/1, Mux6/4
  Demux1/3 -> Mux6/5
  Demux2/3 -> Mux6/7
  Demux1/4 -> Mux1/1
  Demux1/5 -> Mux1/2
  Demux1/6 -> Mux1/3
  Demux1/7 -> Mux1/4
  Demux1/8 -> Mux1/5
  Demux1/9 -> Mux1/6
  Demux1/10 -> Mux1/8
  Demux2/4 -> Mux1/10
  Demux2/5 -> Mux1/11
  Demux2/6 -> Mux1/12
  Demux2/7 -> Mux1/13
  Demux2/8 -> Mux1/14
  Demux2/10 -> Mux1/9
  Demux2/9 -> Mux1/7
  Demux/3 -> beta/1
  Demux/2 -> alpha/1, aerodynamic coefficient/1(a)
  Demux/4 -> "ρ, μ, γ"/1

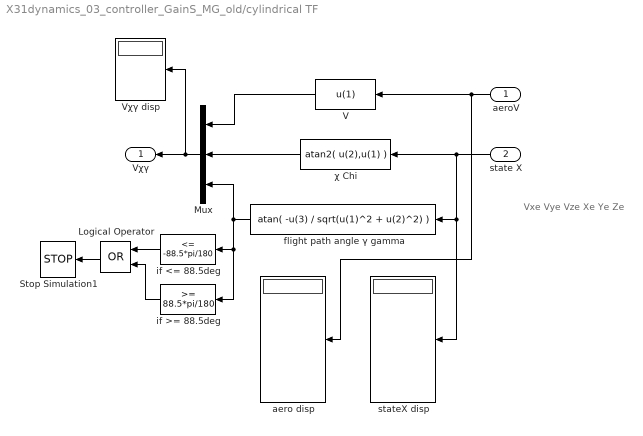
== system X31dynamics_03_controller_GainS_MG_old/cylindrical TF ==
  note: Vxe Vye Vze
      | Xe   Ye   Ze
  aeroV : Inport
  state X : Inport  Port=2
  Logical Operator : Logic  Operator=OR  AllPortsSameDT=off  OutDataTypeStr=boolean
  Mux : Mux  Inputs=3
  Stop Simulation1 : Stop
  V : Fcn  Expr=u(1)
  Vχγ disp : Display
  aero disp : Display
  flight path angle γ gamma : Fcn  Expr=atan( -u(3) / sqrt(u(1)^2 + u(2)^2) )
  if <= 88.5deg : simulink/Logic and Bit Operations/Compare To Constant  relop=<=  const=-88.5*pi/180  OutDataTypeStr=boolean
  if >= 88.5deg : simulink/Logic and Bit Operations/Compare To Constant  relop=>=  const=88.5*pi/180  OutDataTypeStr=boolean
  stateX disp : Display
  χ Chi : Fcn  Expr=atan2( u(2),u(1) )
  Vχγ : Outport
  wires:
  Mux/1 -> Vχγ disp/1, Vχγ/1
  aeroV/1 -> V/1, aero disp/1
  state X/1 -> stateX disp/1, flight path angle γ gamma/1, χ Chi/1
  V/1 -> Mux/1
  χ Chi/1 -> Mux/2
  flight path angle γ gamma/1 -> Mux/3, if >= 88.5deg/1, if <= 88.5deg/1
  if <= 88.5deg/1 -> Logical Operator/1
  if >= 88.5deg/1 -> Logical Operator/2
  Logical Operator/1 -> Stop Simulation1/1

== system X31dynamics_03_controller_GainS_MG_old/geometry(controller) ==
  note: geometric
      |  [Sref, b, Cbar, Xp, Xc, Xr, Xt]
      |
      | Sref : reference wing area
      | b: Wing span
      | Cbar: Mean aerodynamic chord
      | Xp: pilot ahead of c.g.
      | Xc: Canard ahead of c.g.
      | Xr: Rudder aft of c.g.
      | Xt: Engine nozzle after of c.g.
  Cbar : Constant  Value=X31_controller.physical.geometry.Cbar
  Mux6 : Mux  Inputs=7
  Sref : Constant  Value=X31_controller.physical.geometry.Sref
  Xc : Constant  Value=X31_controller.physical.geometry.Xc
  Xp : Constant  Value=X31_controller.physical.geometry.Xp
  Xr : Constant  Value=X31_controller.physical.geometry.Xr
  Xt : Constant  Value=X31_controller.physical.geometry.Xt
  b : Constant  Value=X31_controller.physical.geometry.b
  7 geo param(controller) : Outport
  wires:
  Mux6/1 -> 7 geo param(controller)/1
  Sref/1 -> Mux6/1
  b/1 -> Mux6/2
  Cbar/1 -> Mux6/3
  Xp/1 -> Mux6/4
  Xc/1 -> Mux6/5
  Xr/1 -> Mux6/6
  Xt/1 -> Mux6/7

== system X31dynamics_03_controller_GainS_MG_old/h_rv (4.3.9) ==
  nz_e : Inport
  aero : Inport  Port=2
  Divide : Product  Inputs=*/
  h_rv : Fcn  Expr=1.5 * u(4)/1.23 * ( u(1)/100 )^2
  1 /h_rv : Outport
  wires:
  Divide/1 -> 1 /h_rv/1
  nz_e/1 -> Divide/1
  h_rv/1 -> Divide/2
  aero/1 -> h_rv/1

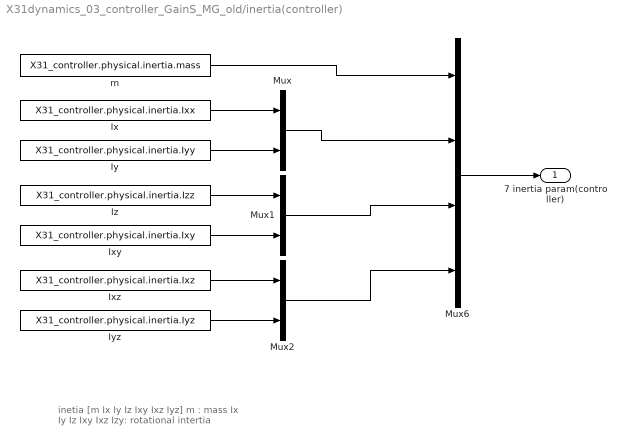
== system X31dynamics_03_controller_GainS_MG_old/inertia(controller) ==
  note: inetia
      | [m Ix Iy Iz Ixy Ixz Iyz]
      | m : mass
      | Ix Iy Iz Ixy Ixz Izy: rotational intertia
  Ix : Constant  Value=X31_controller.physical.inertia.Ixx
  Ixy : Constant  Value=X31_controller.physical.inertia.Ixy
  Ixz : Constant  Value=X31_controller.physical.inertia.Ixz
  Iy : Constant  Value=X31_controller.physical.inertia.Iyy
  Iyz : Constant  Value=X31_controller.physical.inertia.Iyz
  Iz : Constant  Value=X31_controller.physical.inertia.Izz
  Mux : Mux  Inputs=2
  Mux1 : Mux  Inputs=2
  Mux2 : Mux  Inputs=2
  Mux6 : Mux
  m : Constant  Value=X31_controller.physical.inertia.mass
  7 inertia param(controller) : Outport
  wires:
  Ix/1 -> Mux/1
  Iy/1 -> Mux/2
  Ixz/1 -> Mux2/1
  Iyz/1 -> Mux2/2
  Iz/1 -> Mux1/1
  Ixy/1 -> Mux1/2
  Mux6/1 -> 7 inertia param(controller)/1
  m/1 -> Mux6/1
  Mux/1 -> Mux6/2
  Mux1/1 -> Mux6/3
  Mux2/1 -> Mux6/4

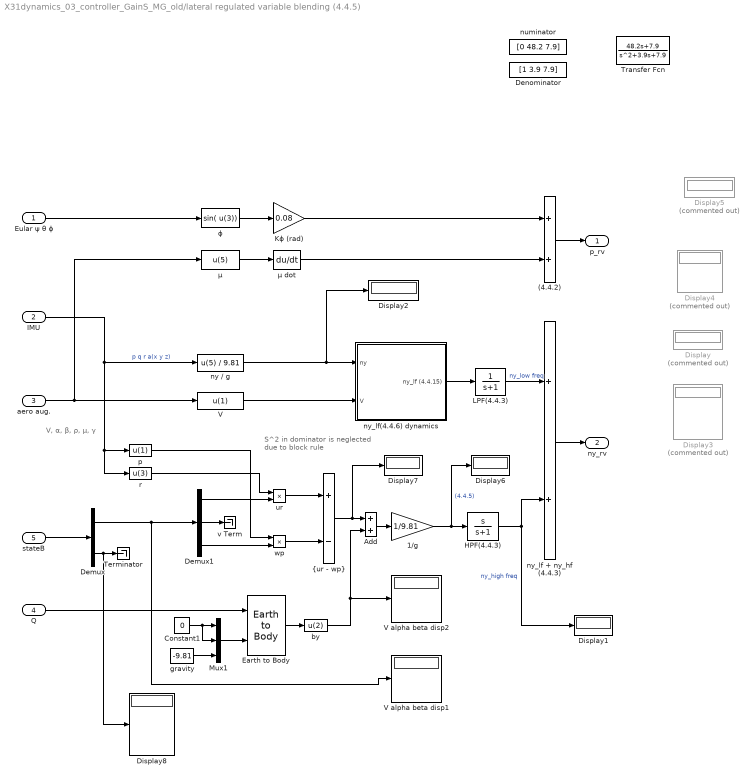
== system X31dynamics_03_controller_GainS_MG_old/lateral regulated variable blending (4.4.5) ==
  note: S^2 in dominator
      | is neglected due to
      | block rule
  note: V, α, β, ρ, μ, γ
  Eular ψ θ ϕ : Inport
  IMU : Inport  Port=2
  aero aug. : Inport  Port=3
  Q : Inport  Port=4
  stateB : Inport  Port=5
  (4.4.2) : Sum
  1/g : Gain  Gain=1/9.81
  Add : Sum
  Constant1 : Constant  Value=0
  Demux : Demux  Outputs=[3 3]
  Demux1 : Demux  Outputs=3
  Denominator : Constant  Value=[1 3.9 7.9]
  Display{,3..5} (4 alike) : Display  Commented=on
  Display{1..2,6..8} (5 alike) : Display
  Earth to Body : QuaternionLib/Earth to Body
  HPF(4.4.3) : TransferFcn  Numerator=[1 0]  Denominator=[1 1]
  Kϕ (rad) : Gain  Gain=0.08
  LPF(4.4.3) : TransferFcn  Denominator=[1 1]
  Mux1 : Mux  Inputs=3
  Terminator : Terminator
  Transfer Fcn : TransferFcn  Numerator=[48.2 7.9]  Denominator=[1 3.9 7.9]
  V : Fcn  Expr=u(1)
  V alpha beta disp1 : Display
  V alpha beta disp2 : Display
  by : Fcn  Expr=u(2)
  gravity : Constant  Value=-9.81
  numinator : Constant  Value=[0 48.2 7.9]
  ny / g : Fcn  Expr=u(5) / 9.81
  ny_lf + ny_hf (4.4.3) : Sum
  ny_lf(4.4.6) dynamics : Subsystem
  p : Fcn  Expr=u(1)
  r : Fcn  Expr=u(3)
  ur : Product
  v Term : Terminator
  wp : Product
  "{ur - wp}" : Sum  Inputs=+-
  μ : Fcn  Expr=u(5)
  μ dot : Derivative
  ϕ : Fcn  Expr=sin( u(3))
  p_rv : Outport
  ny_rv : Outport  Port=2
  wires:
  μ dot/1 -> (4.4.2)/2
  (4.4.2)/1 -> p_rv/1
  LPF(4.4.3)/1 -> ny_lf + ny_hf (4.4.3)/1  "ny_low freq"
  ny_lf + ny_hf (4.4.3)/1 -> ny_rv/1
  Demux/2 -> Display8/1, Terminator/1
  Eular ψ θ ϕ/1 -> ϕ/1
  ϕ/1 -> Kϕ (rad)/1
  Kϕ (rad)/1 -> (4.4.2)/1
  μ/1 -> μ dot/1
  Demux/1 -> Demux1/1, V alpha beta disp1/1
  ur/1 -> "{ur - wp}"/1
  r/1 -> ur/1
  Demux1/1 -> ur/2
  wp/1 -> "{ur - wp}"/2
  p/1 -> wp/1
  Demux1/3 -> wp/2
  Demux1/2 -> v Term/1
  "{ur - wp}"/1 -> Display7/1, Add/1
  Constant1/1 -> Mux1/1, Mux1/2
  gravity/1 -> Mux1/3
  Mux1/1 -> Earth to Body/2
  Q/1 -> Earth to Body/1
  Earth to Body/1 -> by/1
  by/1 -> V alpha beta disp2/1, Add/2
  Add/1 -> 1/g/1
  1/g/1 -> Display6/1, HPF(4.4.3)/1  "(4.4.5)"
  IMU/1 -> p/1, r/1, ny / g/1  "p q r a(x y z)"
  ny / g/1 -> Display2/1, ny_lf(4.4.6) dynamics/1(ny)
  HPF(4.4.3)/1 -> ny_lf + ny_hf (4.4.3)/2, Display1/1  "ny_high freq"
  ny_lf(4.4.6) dynamics/1(ny_lf (4.4.15)) -> LPF(4.4.3)/1
  aero aug./1 -> μ/1, V/1
  V/1 -> ny_lf(4.4.6) dynamics/2(V)
  stateB/1 -> Demux/1

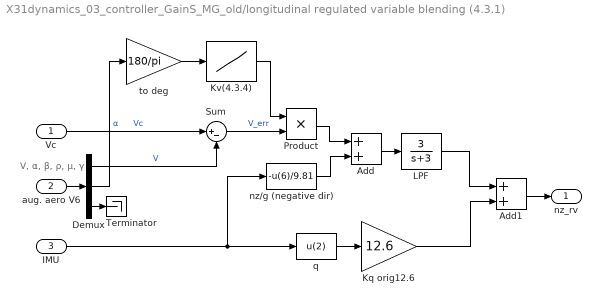
== system X31dynamics_03_controller_GainS_MG_old/longitudinal regulated variable blending (4.3.1) ==
  note: V, α, β, ρ, μ, γ
  Vc : Inport
  aug. aero V6 : Inport  Port=2
  IMU : Inport  Port=3
  Add : Sum
  Add1 : Sum
  Demux : Demux  Outputs=[1 1 4]
  Kq orig12.6 : Gain  Gain=12.6
  Kv(4.3.4) : Lookup_n-D  NumberOfTableDimensions=1  BreakpointsForDimension1=[-85 4.2 32.1 85]  Table=[0.02 0.02 0.15 0.15]  InternalRulePriority=Speed  RndMeth=Simplest  InputSameDT=on
  LPF : TransferFcn  Numerator=[3]  Denominator=[1 3]
  Product : Product
  Sum : Sum  Inputs=|+-
  Terminator : Terminator
  nz/g (negative dir) : Fcn  Expr=-u(6)/9.81
  q : Fcn  Expr=u(2)
  to deg : Gain  Gain=180/pi
  nz_rv : Outport
  wires:
  aug. aero V6/1 -> Demux/1
  q/1 -> Kq orig12.6/1
  IMU/1 -> nz/g (negative dir)/1, q/1
  Vc/1 -> Sum/1  "Vc"
  Demux/1 -> Sum/2  "V"
  nz/g (negative dir)/1 -> Add/2
  Kv(4.3.4)/1 -> Product/1
  Sum/1 -> Product/2  "V_err"
  Product/1 -> Add/1
  Add/1 -> LPF/1
  Kq orig12.6/1 -> Add1/2
  LPF/1 -> Add1/1
  Add1/1 -> nz_rv/1
  to deg/1 -> Kv(4.3.4)/1
  Demux/2 -> to deg/1  "α"
  Demux/3 -> Terminator/1

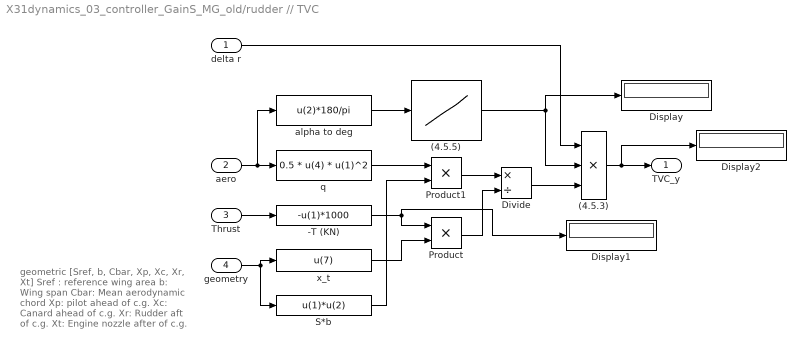
== system X31dynamics_03_controller_GainS_MG_old/rudder // TVC ==
  note: geometric
      |  [Sref, b, Cbar, Xp, Xc, Xr, Xt]
      |
      | Sref : reference wing area
      | b: Wing span
      | Cbar: Mean aerodynamic chord
      | Xp: pilot ahead of c.g.
      | Xc: Canard ahead of c.g.
      | Xr: Rudder aft of c.g.
      | Xt: Engine nozzle after of c.g.
  delta r : Inport
  aero : Inport  Port=2
  Thrust : Inport  Port=3
  geometry : Inport  Port=4
  (4.5.3) : Product  Inputs=3
  (4.5.5) : Lookup_n-D  NumberOfTableDimensions=1  BreakpointsForDimension1=[-85 10 40 85]  Table=[0 0 -0.002 -0.002]  InternalRulePriority=Speed  RndMeth=Simplest  InputSameDT=on
  -T (KN) : Fcn  Expr=-u(1)*1000
  Display : Display
  Display1 : Display
  Display2 : Display
  Divide : Product  Inputs=*/
  Product : Product
  Product1 : Product
  S*b : Fcn  Expr=u(1)*u(2)
  alpha to deg : Fcn  Expr=u(2)*180/pi
  q : Fcn  Expr=0.5 * u(4) * u(1)^2
  x_t : Fcn  Expr=u(7)
  TVC_y : Outport
  wires:
  delta r/1 -> (4.5.3)/1
  aero/1 -> alpha to deg/1, q/1
  geometry/1 -> S*b/1, x_t/1
  Thrust/1 -> -T (KN)/1
  -T (KN)/1 -> Product/1, Display1/1
  x_t/1 -> Product/2
  q/1 -> Product1/1
  S*b/1 -> Product1/2
  Product1/1 -> Divide/1
  Product/1 -> Divide/2
  (4.5.5)/1 -> (4.5.3)/2, Display/1
  Divide/1 -> (4.5.3)/3
  (4.5.3)/1 -> TVC_y/1, Display2/1
  alpha to deg/1 -> (4.5.5)/1

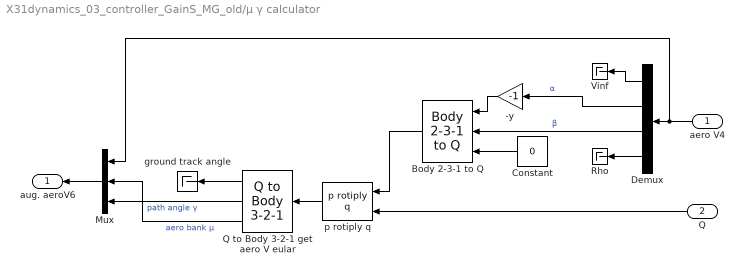
== system X31dynamics_03_controller_GainS_MG_old/μ γ calculator ==
  aero V4 : Inport
  Q : Inport  Port=2
  -y : Gain  Gain=-1
  Body 2-3-1 to Q : QuaternionLib/Body 2-3-1 to Q
  Constant : Constant  Value=0
  Demux : Demux  Outputs=[1 1 1 1]
  Mux : Mux  Inputs=3
  Q to Body 3-2-1 get aero V eular : QuaternionLib/Q to Body 3-2-1
  Rho : Terminator
  Vinf : Terminator
  ground track angle : Terminator
  p rotiply q : QuaternionLib/p rotiply q
  aug. aeroV6 : Outport
  wires:
  Q/1 -> p rotiply q/2
  Demux/1 -> Vinf/1
  Demux/4 -> Rho/1
  Demux/2 -> -y/1  "α"
  Demux/3 -> Body 2-3-1 to Q/2  "β"
  aero V4/1 -> Mux/1, Demux/1
  -y/1 -> Body 2-3-1 to Q/1
  Constant/1 -> Body 2-3-1 to Q/3
  Body 2-3-1 to Q/1 -> p rotiply q/1
  p rotiply q/1 -> Q to Body 3-2-1 get aero V eular/1
  Mux/1 -> aug. aeroV6/1
  Q to Body 3-2-1 get aero V eular/1 -> ground track angle/1
  Q to Body 3-2-1 get aero V eular/2 -> Mux/3  "path angle γ"
  Q to Body 3-2-1 get aero V eular/3 -> Mux/2  "aero bank μ"

== system X31dynamics_03_controller_GainS_MG_old/ψ θ ϕ calculator ==
  Q : Inport
  Mux : Mux  Inputs=3
  Q to Body 3-2-1 : QuaternionLib/Q to Body 3-2-1
  Eular ψ θ ϕ : Outport
  wires:
  Q/1 -> Q to Body 3-2-1/1
  Mux/1 -> Eular ψ θ ϕ/1
  Q to Body 3-2-1/1 -> Mux/1  "ψ: heading angle"
  Q to Body 3-2-1/2 -> Mux/2  "θ: pitch angle"
  Q to Body 3-2-1/3 -> Mux/3  "ϕ : body bank angle"

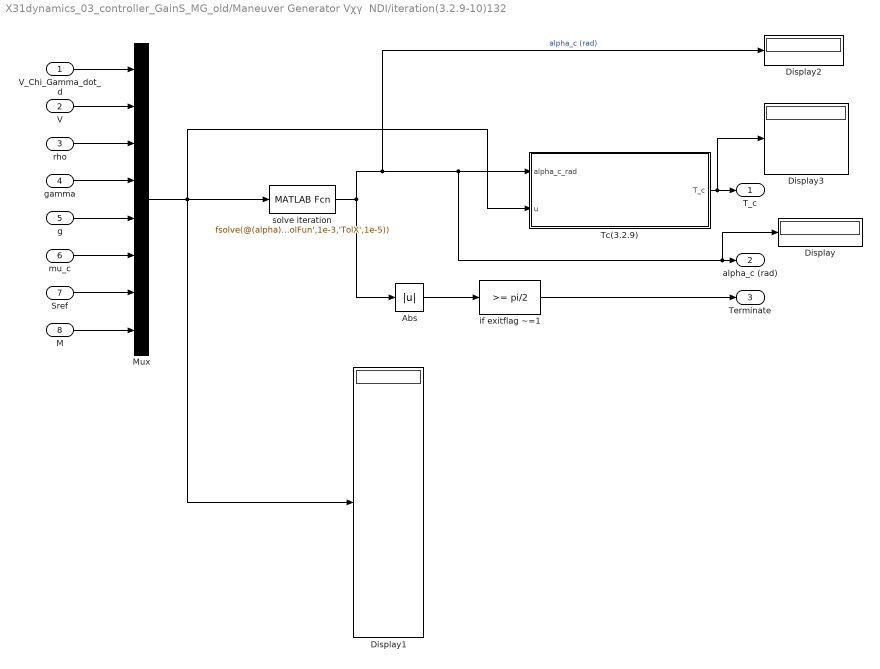
== system X31dynamics_03_controller_GainS_MG_old/Maneuver Generator Vχγ  NDI/iteration(3.2.9-10)132 ==
  V_Chi_Gamma_dot_d : Inport
  V : Inport  Port=2
  rho : Inport  Port=3
  gamma : Inport  Port=4
  g : Inport  Port=5
  mu_c : Inport  Port=6
  Sref : Inport  Port=7
  M : Inport  Port=8
  Abs : Abs
  Display{,1..3} (4 alike) : Display
  Mux : Mux  Inputs=8
  Tc(3.2.9) : MATLAB Function  TreatAsAtomicUnit=on
  if exitflag ~=1 : simulink/Logic and Bit Operations/Compare To Constant  relop=>=  const=pi/2  OutDataTypeStr=boolean
  solve iteration : MATLABFcn  MATLABFcn="fsolve(@(alpha)X31dynamics_03_controller_MG_iter_3_2_9_10(alpha, u(1),u(2), u(3), u(4), u(5),u(6), u(7), u(8), u(9), u(10) ),  2, optimset('Display','off', 'TolFun',1e-3,'TolX',1e-5))"
  T_c : Outport
  alpha_c (rad) : Outport  Port=2
  Terminate : Outport  Port=3
  wires:
  V_Chi_Gamma_dot_d/1 -> Mux/1
  V/1 -> Mux/2
  rho/1 -> Mux/3
  gamma/1 -> Mux/4
  g/1 -> Mux/5
  mu_c/1 -> Mux/6
  Sref/1 -> Mux/7
  M/1 -> Mux/8
  Mux/1 -> Display1/1, solve iteration/1, Tc(3.2.9)/2(u)
  solve iteration/1 -> Display2/1, Display/1, alpha_c (rad)/1, Tc(3.2.9)/1(alpha_c_rad), Abs/1  "alpha_c (rad)"
  if exitflag ~=1/1 -> Terminate/1
  Tc(3.2.9)/1(T_c) -> Display3/1, T_c/1
  Abs/1 -> if exitflag ~=1/1

== system X31dynamics_03_controller_GainS_MG_old/Maneuver Generator Vχγ  NDI/μc (3.2.7) ==
  V : Inport
  χ dot des : Inport  Port=2
  γ dot des : Inport  Port=3
  γ : Inport  Port=4
  g : Inport  Port=5
  Mux : Mux  Inputs=5
  μ1c : Fcn  Expr="atan2(  u(1)*u(2)*cos(u(4)) , (u(1)*u(3) + u(5)*cos(u(4)))  )"
  μc : Outport
  wires:
  V/1 -> Mux/1
  χ dot des/1 -> Mux/2
  γ dot des/1 -> Mux/3
  g/1 -> Mux/5
  Mux/1 -> μ1c/1
  μ1c/1 -> μc/1
  γ/1 -> Mux/4

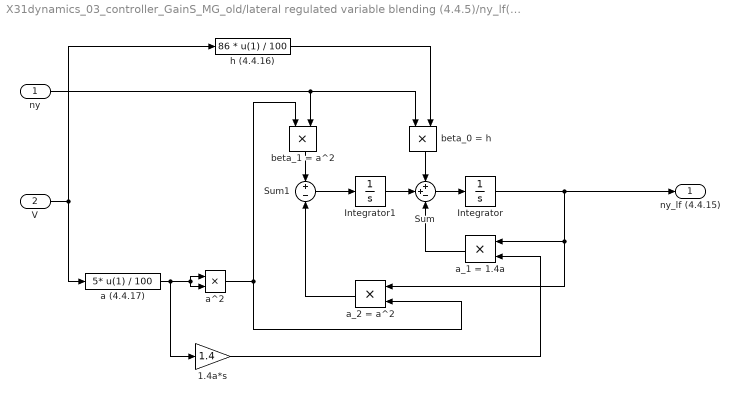
== system X31dynamics_03_controller_GainS_MG_old/lateral regulated variable blending (4.4.5)/ny_lf(4.4.6) dynamics ==
  ny : Inport
  V : Inport  Port=2
  1.4a*s : Gain  Gain=1.4
  Integrator : Integrator
  Integrator1 : Integrator
  Sum : Sum  Inputs=++-
  Sum1 : Sum  Inputs=+-
  a (4.4.17) : Fcn  Expr=5* u(1) / 100
  a^2 : Product
  a_1 = 1.4a : Product
  a_2 = a^2 : Product
  beta_0 = h : Product
  beta_1 = a^2 : Product
  h (4.4.16) : Fcn  Expr=86 * u(1) / 100
  ny_lf (4.4.15) : Outport
  wires:
  Sum/1 -> Integrator/1
  Sum1/1 -> Integrator1/1
  Integrator1/1 -> Sum/2
  ny/1 -> beta_0 = h/1, beta_1 = a^2/2
  h (4.4.16)/1 -> beta_0 = h/2
  a (4.4.17)/1 -> 1.4a*s/1, a^2/1, a^2/2
  1.4a*s/1 -> a_1 = 1.4a/2
  V/1 -> a (4.4.17)/1, h (4.4.16)/1
  beta_1 = a^2/1 -> Sum1/1
  a^2/1 -> beta_1 = a^2/1, a_2 = a^2/2
  beta_0 = h/1 -> Sum/1
  Integrator/1 -> a_2 = a^2/1, a_1 = 1.4a/1, ny_lf (4.4.15)/1
  a_1 = 1.4a/1 -> Sum/3
  a_2 = a^2/1 -> Sum1/2

== matlab function X31dynamics_03_controller_GainS_MG_old/coefficient/aerodynamic coefficient ==
  data: fa output; a input; fb output; X31_initP parameter
function [fa,fb] = aero_coef(a,X31_initP)
    fa = zeros(1,10);
    fb = zeros(1,10);
    a = 180 / pi * a;   % convert to degree for polynomials
    a_abs = abs(a);
    for i = 1:10
        fa(i) = X31_initP.fig2_2(i).a(6)*a_abs^6 + X31_initP.fig2_2(i).a(5)*a_abs^5 + X31_initP.fig2_2(i).a(4)*a_abs^4 +...
                X31_initP.fig2_2(i).a(3)*a_abs^3 + X31_initP.fig2_2(i).a(2)*a_abs^2 + X31_initP.fig2_2(i).a(1)*a_abs + X31_initP.fig2_2(i).a(7);

        fb(i) = X31_initP.fig2_2(i).b(6)*a_abs^6 + X31_initP.fig2_2(i).b(5)*a_abs^5 + X31_initP.fig2_2(i).b(4)*a_abs^4 +...
                X31_initP.fig2_2(i).b(3)*a_abs^3 + X31_initP.fig2_2(i).b(2)*a_abs^2 + X31_initP.fig2_2(i).b(1)*a_abs + X31_initP.fig2_2(i).b(7);
        % for odd functions
        if (a<0) 
            if (X31_initP.fig2_2(i).a(8) ==1)
                fa(i) = -fa(i) + 2*X31_initP.fig2_2(i).a(7);
            end
            if (X31_initP.fig2_2(i).b(8) ==1)
                fb(i) = -fb(i) + 2*X31_initP.fig2_2(i).b(7);
            end
        end
    end
end

%{
     Force
CL   (α) 2.2.1a Odd
CLdc (α) 2.2.2a Even
C0d  (α) 2.2.2/l0b Odd
CD   (α) 2.2.1b Even
CYp  (α) 2.2.3a Even
CYda (α) Set zero Not Shown Even
CYdr (α) 2.2.3b Even

     Moment
Clb  (α) 2.2.4a Even
Clp  (α) 2.2.5a Even
Clr  (α) 2.2.6a Odd
Clda (α) 2.2.7a Even
Cldr (α) 2.2.8a Even

Cm0  (α) 4.65% e unstable 2.2.9a Odd
Cmq  (α) 3 2.2.9b Even
Cmdc      2.2.10a Even
C0d  (α) 2.2.2/10b Odd

Cnb  (α) 2.2.4b Even
Cnp  (α) 2.2.5b Odd
Cnr  (α) 2.2.6b Even
Cnda (α) 2.2.7b Even
Cndr (α) 2.2.8b Even
%}

== matlab function X31dynamics_03_controller_GainS_MG_old/Maneuver Generator Vχγ  NDI/iteration(3.2.9-10)132/Tc(3.2.9) ==
  data: alpha_c_rad input; u input; T_c output; X31_controller parameter
function T_c = Tc_from_alpha_C(alpha_c_rad, u, X31_controller)
V_dot_d = u(1);
V = u(4);
rho = u(5);
gamma = u(6);
g = u(7);
Sref = u(9);
M = u(10);

% Drag
alpha_c_deg = 180 / pi * alpha_c_rad;   % convert to degree for polynomials
a_abs = abs(alpha_c_deg);

fig2_2_1b = X31_controller.aero_poly.fig2_2(1).b;
      % figer 2.2.1b is the Drag coefficient
CD = fig2_2_1b(6)*a_abs^6 + fig2_2_1b(5)*a_abs^5 + fig2_2_1b(4)*a_abs^4 +...
                fig2_2_1b(3)*a_abs^3 + fig2_2_1b(2)*a_abs^2 + fig2_2_1b(1)*a_abs + fig2_2_1b(7);
Drag = 0.5*rho*V^2*Sref*CD;

T_c = 1/cos(alpha_c_rad) * (M*V_dot_d + Drag + M*g*sin(gamma));
end
